simulink model "main"  (R2017b)
settings: Solver=FixedStepAuto  StartTime=0.0  StopTime=60  FixedStep=Ts  RelTol=1e-3
values from neighbouring files (symbols this model uses):
  ekfPendel = observer.formParameters()    [prepareWorkspace.m]
  Ts = 0.005    [prepareWorkspace.m]
undefined symbols (not defined in the file or in its folder): lambda, sigma, w0
libraries: hydro x2
settings Model: Creator=motionlab  LastModifiedBy=motionlab
settings OptimizationCC: LocalBlockOutputs=off
settings DebuggingCC: BusObjectLabelMismatch=error
settings SFSimCC: SimCustomHeaderCode=|
  | #include <ioTypes.h>
  | #include <simTypes.h>
  | #include <plcTypes.h>
settings RTWCC: SystemTargetFile=TwinCAT.tlc  GenCodeOnly=on  MakeCommand=make_tct  TemplateMakefile=tct_msbuild.tmf  Description=TwinCAT Target  GenerateReport=on  TargetLang=C++
settings STFCustomTargetCC: TargetLangStandard=C++03 (ISO)  CompOptLevelCompliant=on  MATLABClassNameForMDSCustomization=Simulink.SoftwareTarget.TargetSpecificTriggerConfigurationBase  SystemTargetFile=TwinCAT.tlc

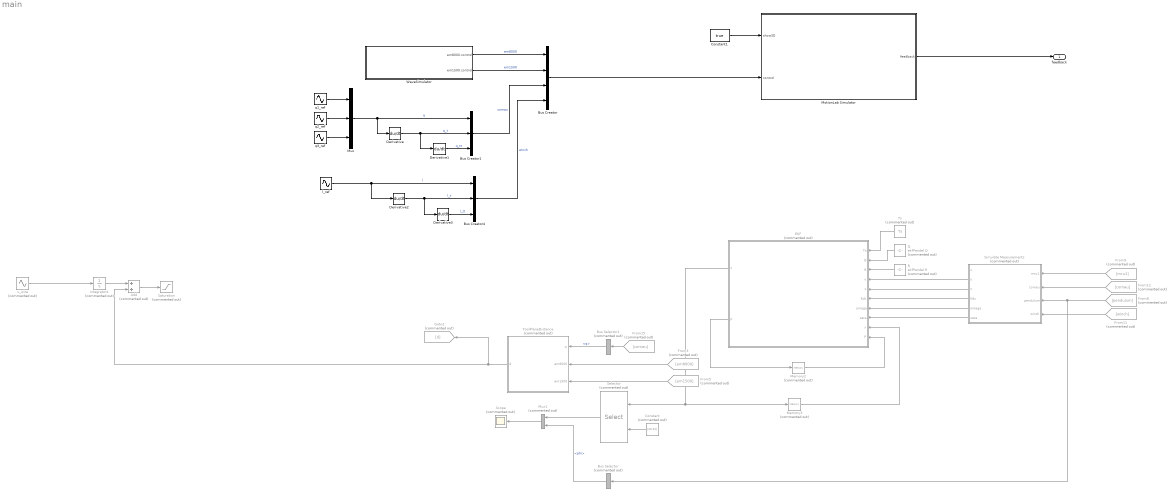
== system main ==
  Add : Sum  Commented=on
  Bus Creator : BusCreator  Inputs=4  OutDataTypeStr=Bus: ST_Control
  Bus Creator1 : BusCreator  Inputs=3  OutDataTypeStr=Bus: ST_ComauControl
  Bus Creator4 : BusCreator  Inputs=3  OutDataTypeStr=Bus: ST_WinchControl
  Bus Selector : BusSelector  Commented=on  OutputSignals=phi
  Bus Selector1 : BusSelector  Commented=on  OutputSignals=q
  Constant : Constant  Commented=on  Value=[30:31]
  Constant1 : Constant  Value=true
  Derivative{,1..3} (4 alike) : Derivative
  EKF : MATLAB Function  Commented=on  TreatAsAtomicUnit=on
  From11 : From  Commented=on  GotoTag=winch
  From12 : From  Commented=on  GotoTag=comau
  From15 : From  Commented=on  GotoTag=comau
  From3 : From  Commented=on  GotoTag=em8000
  From5 : From  Commented=on  GotoTag=em1500
  From8 : From  Commented=on  GotoTag=pendulum
  From9 : From  Commented=on  GotoTag=mru1
  Goto2 : Goto  Commented=on  GotoTag=d
  Integrator4 : Integrator  Commented=on
  Memory2 : Memory  Commented=on  InitialCondition=ekfPendel.P
  Memory3 : Memory  Commented=on  InitialCondition=ekfPendel.x0
  MotionLab Simulator : Subsystem
  Mux : Mux  Inputs=3
  Mux1 : Mux  Commented=on  Inputs=2
  Q : Constant  Commented=on  Value=ekfPendel.Q
  R : Constant  Commented=on  Value=ekfPendel.R
  Saturation : Saturate  Commented=on  UpperLimit=4.0  LowerLimit=0.5
  Scope : Scope  Commented=on
  Selector : Selector  Commented=on  InputPortWidth=34  IndexOptions=Index vector (port)  Indices=[1 3]  OutputSizes=1
  Simulate Measurements : MATLAB Function  Commented=on  TreatAsAtomicUnit=on
  ToolPlaneDistance : Subsystem  Commented=on  mask{d=-0.5}
      mask prompts: d "Plane-BodyOrigo Distance"
  Ts : Constant  Commented=on  Value=Ts
  WaveSimulator : Subsystem  mask{w0=w0, sigma=sigma, lambda=lambda}
      mask prompts: w0 "Peak Frequency"; sigma "Wave Intensity"; lambda "Damping"
  l_ref : Sin  Amplitude=0  Bias=2  Frequency=0.2*2*pi  SampleTime=0
  q1_ref : Sin  Amplitude=10/180*pi  Frequency=0.2*2*pi  SampleTime=0
  q2_ref : Sin  Amplitude=0  Frequency=0.1*2*pi  SampleTime=0
  q3_ref : Sin  Amplitude=0  Bias=-pi/2  Frequency=0.12*2*pi  SampleTime=0
  v_wire : Sin  Commented=on  Amplitude=0  Frequency=0.2*2*pi  SampleTime=0
  feedback : Outport
  wires:
  q2_ref/1 -> Mux/2
  q3_ref/1 -> Mux/3
  Mux/1 -> Bus Creator1/1, Derivative/1  "q"
  Derivative/1 -> Derivative1/1, Bus Creator1/2  "q_t"
  q1_ref/1 -> Mux/1
  Add/1 -> Saturation/1
  Integrator4/1 -> Add/1
  v_wire/1 -> Integrator4/1
  From3/1 -> ToolPlaneDistance/2(em8000)
  From5/1 -> ToolPlaneDistance/3(em1500)
  ToolPlaneDistance/1(d) -> Goto2/1, Add/2
  From12/1 -> Simulate Measurements/2(comau)
  From11/1 -> Simulate Measurements/4(winch)
  From9/1 -> Simulate Measurements/1(mru1)
  Ts/1 -> EKF/1(Ts)
  R/1 -> EKF/3(R)
  Simulate Measurements/6(zeta) -> EKF/8(zeta)
  Simulate Measurements/3(z) -> EKF/5(z)
  EKF/1(x) -> Memory3/1, Selector/1
  Memory3/1 -> EKF/9("x ")
  Q/1 -> EKF/2(Q)
  Simulate Measurements/2(u) -> EKF/4(u)
  Simulate Measurements/4(Kdc) -> EKF/6(Kdc)
  Memory2/1 -> EKF/10("P ")
  Selector/1 -> Mux1/1
  From8/1 -> Bus Selector/1, Simulate Measurements/3(pendulum)
  Simulate Measurements/5(omega) -> EKF/7(omega)
  Constant/1 -> Selector/2
  Mux1/1 -> Scope/1
  EKF/2(P) -> Memory2/1
  Bus Selector/1 -> Mux1/2  "<phi>"
  From15/1 -> Bus Selector1/1
  Bus Selector1/1 -> ToolPlaneDistance/1(q)  "<q>"
  Derivative1/1 -> Bus Creator1/3  "q_tt"
  Derivative2/1 -> Derivative3/1, Bus Creator4/2  "l_t"
  Derivative3/1 -> Bus Creator4/3  "l_tt"
  l_ref/1 -> Derivative2/1, Bus Creator4/1  "l"
  WaveSimulator/1(em8000.control) -> Bus Creator/1  "em8000"
  WaveSimulator/2(em1500.control) -> Bus Creator/2  "em1500"
  Bus Creator1/1 -> Bus Creator/3  "comau"
  Bus Creator4/1 -> Bus Creator/4  "winch"
  Bus Creator/1 -> MotionLab Simulator/2(control)
  MotionLab Simulator/1(feedback) -> feedback/1
  Constant1/1 -> MotionLab Simulator/1(show3D)

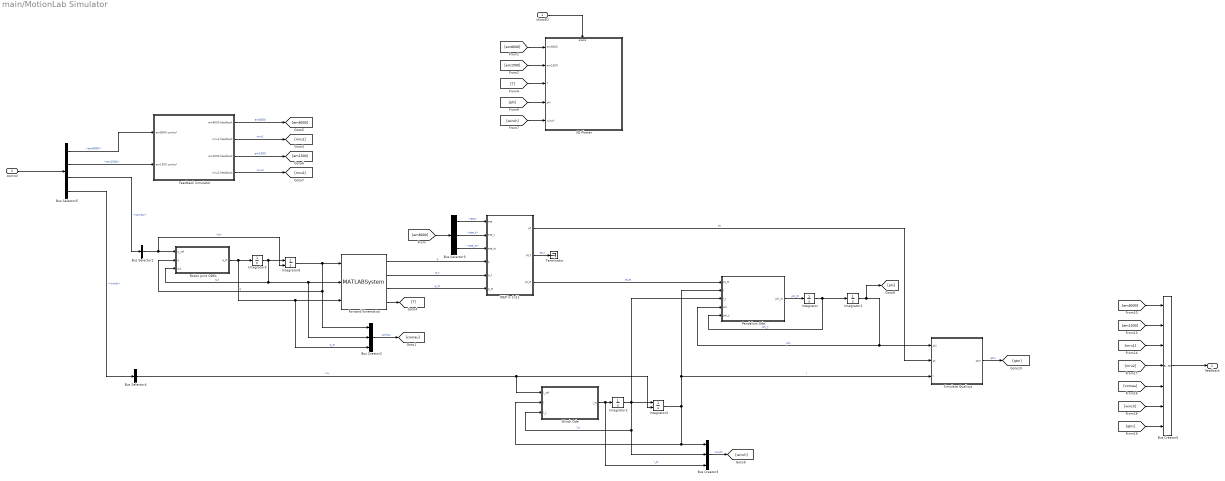
== system main/MotionLab Simulator ==
  show3D : Inport
  control : Inport  Port=2
  3D Plotter : Subsystem
  Bus Creator2 : BusCreator  Inputs=3  OutDataTypeStr=Bus: ST_ComauFeedback
  Bus Creator3 : BusCreator  Inputs=3  OutDataTypeStr=Bus: ST_WinchFeedback
  Bus Creator5 : BusCreator  Inputs=7  OutDataTypeStr=Bus: ST_Feedback
  Bus Selector2 : BusSelector  OutputSignals=q
  Bus Selector3 : BusSelector  OutputSignals=eta,eta_t,eta_tt
  Bus Selector4 : BusSelector  OutputSignals=l
  Bus Selector5 : BusSelector  OutputSignals=em8000,em1500,comau,winch
  Feedback Simulator : Subsystem
  Forward Kinematics : MATLABSystem  System=motionlab.ComauRobot3DOF  dt=L  fk=on  outputT=on  SimulateUsing=Interpreted execution
      mask Type: motionlab.ComauRobot3DOF
      mask Display:
      | disp('ComauRobot3DOF');
      | port_label('input',1,'q');
      | port_label('input',2,'q_t');
      | port_label('input',3,'q_tt');
      | port_label('output',1,'p');
      | port_label('output',2,'p_t');
      | port_label('output',3,'p_tt');
      | port_label('output',4,'T');
  Integrator : Integrator  InitialCondition=zeros(2,1)
  Integrator1 : Integrator  InitialCondition=zeros(2,1)
  Integrator2 : Integrator
  Integrator3 : Integrator  InitialConditionSource=external
  Integrator5 : Integrator  InitialCondition=zeros(3,1)
  Integrator6 : Integrator  InitialConditionSource=external  InitialCondition=zeros(3,1)
  Pendelum Ode : MATLAB Function  TreatAsAtomicUnit=on  SystemSampleTime=Ts
  Robot Joint ODEs : MATLAB Function  TreatAsAtomicUnit=on
  Simulate Qualisys : MATLAB Function  TreatAsAtomicUnit=on
  Terminator : Terminator
  "WEP in {n1}" : MATLAB Function  TreatAsAtomicUnit=on
  Winch Ode : MATLAB Function  TreatAsAtomicUnit=on
  feedback : Outport
  wires:
  [mru1] -> Bus Creator5/3
  [winch] -> 3D Plotter/5(winch)
  [mru2] -> Bus Creator5/4
  [em1500] -> Bus Creator5/2
  [em8000] -> Bus Creator5/1
  Bus Creator3/1 -> [winch]  "winch"
  Bus Creator5/1 -> feedback/1
  [qtm] -> Bus Creator5/7
  [comau] -> Bus Creator5/5
  [winch] -> Bus Creator5/6
  "WEP in {n1}"/2(pt_t) -> Terminator/1  "pt_t"
  Winch Ode/1(l_tt) -> Bus Creator3/3, Integrator2/1  "l_tt"
  show3D/1 -> 3D Plotter/Enable
  Integrator/1 -> Integrator1/1, Pendelum Ode/5(phi_t)  "phi_t"
  "WEP in {n1}"/3(pt_tt) -> Pendelum Ode/1(pt_tt)  "pt_tt"
  Forward Kinematics/4 -> [T]
  Bus Selector2/1 -> Robot Joint ODEs/1(q_ref), Integrator6/2  "<q>"
  Pendelum Ode/1(phi_tt) -> Integrator/1  "phi_tt"
  Integrator3/1 -> Winch Ode/2(l), Bus Creator3/1, Pendelum Ode/2(l), Simulate Qualisys/3(l)  "l"
  Integrator2/1 -> Pendelum Ode/3(l_t), Bus Creator3/2, Winch Ode/3(l_t), Integrator3/1  "l_t"
  Integrator1/1 -> [phi], Pendelum Ode/4(phi), Simulate Qualisys/1(phi)  "phi"
  Robot Joint ODEs/1(q_tt) -> Integrator5/1, Bus Creator2/3, Forward Kinematics/3  "q_tt"
  Integrator5/1 -> Robot Joint ODEs/3(q_t), Forward Kinematics/2, Bus Creator2/2, Integrator6/1  "q_t"
  Integrator6/1 -> Bus Creator2/1, Robot Joint ODEs/2(q), Forward Kinematics/1  "q"
  Forward Kinematics/1 -> "WEP in {n1}"/4(p)  "p"
  Forward Kinematics/2 -> "WEP in {n1}"/5(p_t)  "p_t"
  Forward Kinematics/3 -> "WEP in {n1}"/6(p_tt)  "p_tt"
  Simulate Qualisys/1(qtm) -> [qtm]  "qtm"
  Bus Selector4/1 -> Winch Ode/1(l_ref), Integrator3/2  "<l>"
  control/1 -> Bus Selector5/1
  Bus Selector5/1 -> Feedback Simulator/1(em8000.control)  "<em8000>"
  Bus Selector3/1 -> "WEP in {n1}"/1(eta)  "<eta>"
  Bus Selector3/3 -> "WEP in {n1}"/3(eta_tt)  "<eta_tt>"
  Bus Selector3/2 -> "WEP in {n1}"/2(eta_t)  "<eta_t>"
  "WEP in {n1}"/1(pt) -> Simulate Qualisys/2(pt)  "pt"
  Bus Selector5/2 -> Feedback Simulator/2(em1500.control)  "<em1500>"
  Feedback Simulator/1(em8000.feedback) -> [em8000]  "em8000"
  [phi] -> 3D Plotter/4(phi)
  Feedback Simulator/3(em1500.feedback) -> [em1500]  "em1500"
  [em8000] -> Bus Selector3/1
  [em1500] -> 3D Plotter/2(em1500)
  Feedback Simulator/2(mru1.feedback) -> [mru1]  "mru1"
  Bus Selector5/3 -> Bus Selector2/1  "<comau>"
  [em8000] -> 3D Plotter/1(em8000)
  Bus Creator2/1 -> [comau]  "comau"
  Feedback Simulator/4(mru2.feedback) -> [mru2]  "mru2"
  Bus Selector5/4 -> Bus Selector4/1  "<winch>"
  [T] -> 3D Plotter/3(T)

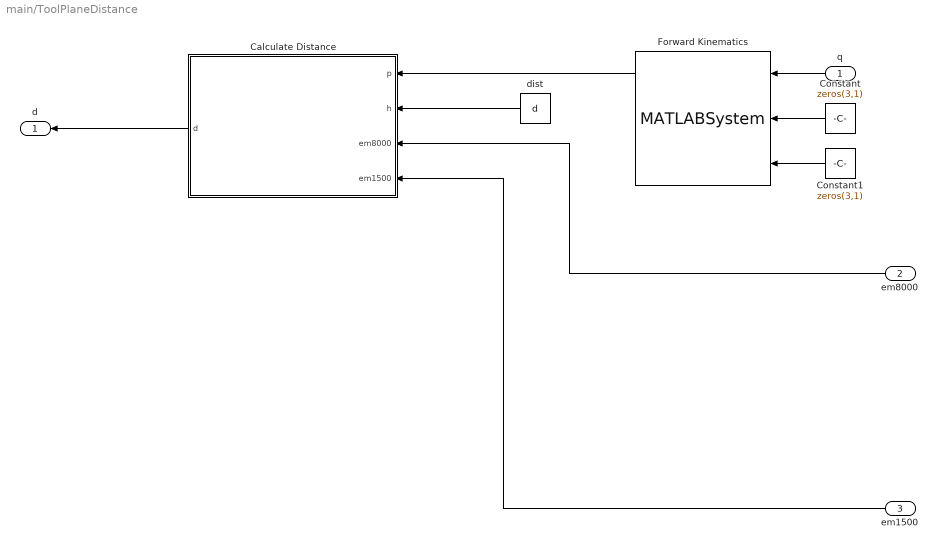
== system main/ToolPlaneDistance ==
  q : Inport
  em8000 : Inport  Port=2  OutDataTypeStr=Bus: StewartFeedback
  em1500 : Inport  Port=3  OutDataTypeStr=Bus: StewartFeedback
  Calculate Distance : MATLAB Function  TreatAsAtomicUnit=on
  Constant : Constant  Value=zeros(3,1)
  Constant1 : Constant  Value=zeros(3,1)
  Forward Kinematics : MATLABSystem  System=motionlab.ComauRobot3DOF  dt=L  fk=on  outputT=off  SimulateUsing=Interpreted execution
      mask Type: motionlab.ComauRobot3DOF
      mask Display:
      | disp('ComauRobot3DOF');
      | port_label('input',1,'q');
      | port_label('input',2,'q_t');
      | port_label('input',3,'q_tt');
      | port_label('output',1,'p');
      | port_label('output',2,'p_t');
      | port_label('output',3,'p_tt');
  dist : Constant  Value=d
  d : Outport
  wires:
  Calculate Distance/1(d) -> d/1
  Constant/1 -> Forward Kinematics/2
  Constant1/1 -> Forward Kinematics/3
  dist/1 -> Calculate Distance/2(h)
  em1500/1 -> Calculate Distance/4(em1500)
  em8000/1 -> Calculate Distance/3(em8000)
  Forward Kinematics/1 -> Calculate Distance/1(p)
  q/1 -> Forward Kinematics/1

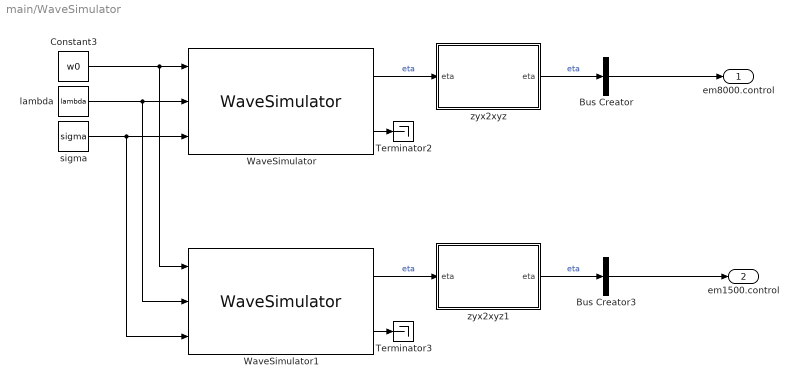
== system main/WaveSimulator ==
  Bus Creator : BusCreator  Inputs=1  OutDataTypeStr=Bus: ST_StewartControl
  Bus Creator3 : BusCreator  Inputs=1  OutDataTypeStr=Bus: ST_StewartControl
  Constant3 : Constant  Value=w0
  Terminator2 : Terminator
  Terminator3 : Terminator
  WaveSimulator : hydro/WaveSimulator  poles=-30  seed=[0,20,510,9000,400,200]  K1=1e4  K2=1e4  K3=1e8  K4=1e7  K5=1e8  K6=1e3  maxOutput=[0.2, 0.2, 0.4, 10/180*pi, 10/180*pi, 5/180*pi]  limitK=[1, 1, 0.15, 1, 1, 1]
      settings: SourceProductName=Hydro Library
  WaveSimulator1 : hydro/WaveSimulator  poles=-30  seed=[5000,400,0,9000,150,42]  K1=1e4  K2=1e4  K3=1e8  K4=1e7  K5=1e8  K6=1e3  maxOutput=[0.2, 0.2, 0.4, 5/180*pi, 5/180*pi, 5/180*pi]  limitK=[1, 1, 0.15, 1, 1, 1]
      settings: SourceProductName=Hydro Library
  lambda : Constant  Value=lambda
  sigma : Constant  Value=sigma
  zyx2xyz : MATLAB Function  TreatAsAtomicUnit=on
  zyx2xyz1 : MATLAB Function  TreatAsAtomicUnit=on
  em8000.control : Outport
  em1500.control : Outport  Port=2
  wires:
  zyx2xyz/1(eta) -> Bus Creator/1  "eta"
  Bus Creator3/1 -> em1500.control/1
  Bus Creator/1 -> em8000.control/1
  zyx2xyz1/1(eta) -> Bus Creator3/1  "eta"
  sigma/1 -> WaveSimulator1/3, WaveSimulator/3
  Constant3/1 -> WaveSimulator1/1, WaveSimulator/1
  WaveSimulator1/1 -> zyx2xyz1/1("eta ")  "eta"
  WaveSimulator/2 -> Terminator2/1
  WaveSimulator/1 -> zyx2xyz/1("eta ")  "eta"
  lambda/1 -> WaveSimulator1/2, WaveSimulator/2
  WaveSimulator1/2 -> Terminator3/1

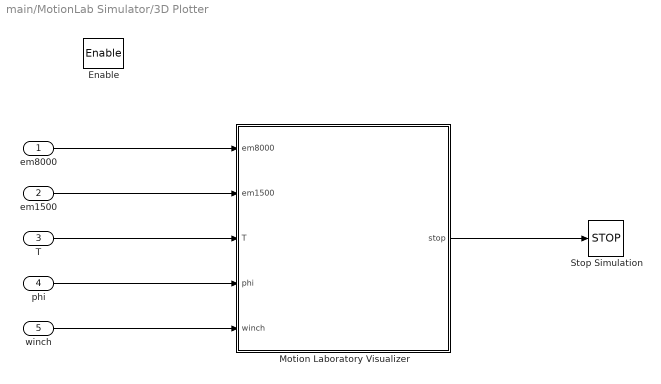
== system main/MotionLab Simulator/3D Plotter ==
  em8000 : Inport
  em1500 : Inport  Port=2
  T : Inport  Port=3
  phi : Inport  Port=4
  winch : Inport  Port=5
  Enable : EnablePort
  Motion Laboratory Visualizer : MATLAB Function  TreatAsAtomicUnit=on  SystemSampleTime=0.1
  Stop Simulation : Stop
  wires:
  em8000/1 -> Motion Laboratory Visualizer/1(em8000)
  phi/1 -> Motion Laboratory Visualizer/4(phi)
  winch/1 -> Motion Laboratory Visualizer/5(winch)
  em1500/1 -> Motion Laboratory Visualizer/2(em1500)
  T/1 -> Motion Laboratory Visualizer/3(T)
  Motion Laboratory Visualizer/1(stop) -> Stop Simulation/1

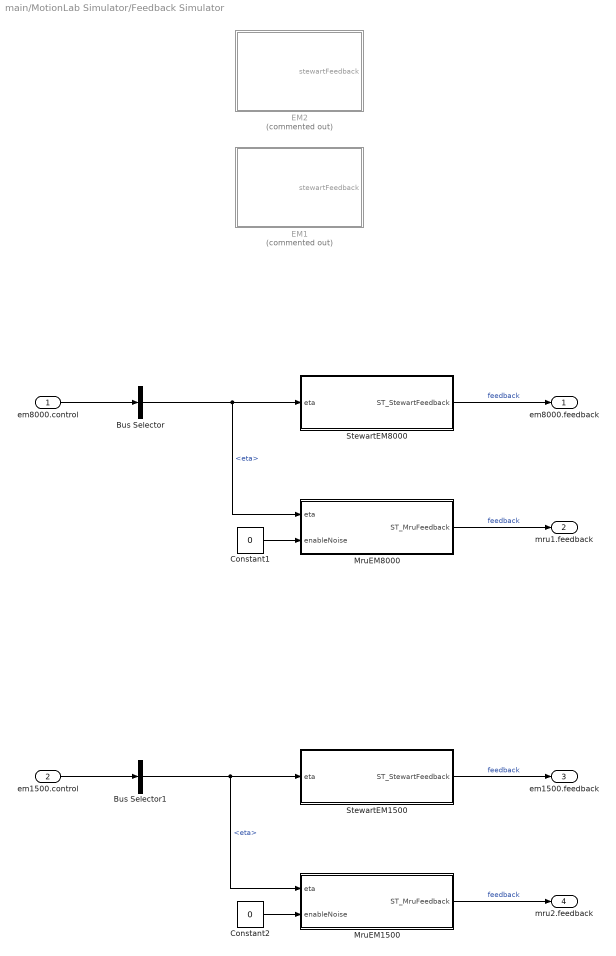
== system main/MotionLab Simulator/Feedback Simulator ==
  em8000.control : Inport  OutDataTypeStr=Bus: ST_StewartControl
  em1500.control : Inport  Port=2  OutDataTypeStr=Bus: ST_StewartControl
  Bus Selector : BusSelector  OutputSignals=eta
  Bus Selector1 : BusSelector  OutputSignals=eta
  Constant1 : Constant  Value=0
  Constant2 : Constant  Value=0
  EM1 : Subsystem  Commented=on  TreatAsAtomicUnit=on  mask{A_surge=0.2, f_surge=0.1, phase_surge=0, A_sway=0.2, f_sway=0.05, phase_sway=200, A_heave=0.4, f_heave=0.12, phase_heave=30, A_phi=5.0, f_phi=0.09, phase_phi=45, A_theta=5.0, f_theta=0.15, phase_theta=60, A_psi=5.0, f_psi=0.12, phase_psi=-40}
      mask prompts: A_surge "Amplitude [m]"; f_surge "Frequency [Hz]"; phase_surge "Phase [deg]"; A_sway "Amplitude [m]"; f_sway "Frequency [Hz]"; phase_sway "Phase [deg]"; A_heave "Amplitude [m]"; f_heave "Frequency [Hz]"; phase_heave "Phase [deg]"; A_phi "Amplitude [deg]"; f_phi "Frequency [Hz]"; phase_phi "Phase [deg]"; A_theta "Amplitude [deg]"; f_theta "Frequency [Hz]"; phase_theta "Phase [deg]"; A_psi "Amplitude [deg]"; f_psi "Frequency [Hz]"; phase_psi "Phase [deg]"
      mask DialogControl ParameterGroupVar Prompt: Surge
      mask DialogControl Container3 Prompt: Sway
      mask DialogControl Container4 Prompt: Heave
      mask DialogControl Container5 Prompt: Phi
      mask DialogControl Container6 Prompt: Theta
      mask DialogControl Container7 Prompt: Psi
  EM2 : Subsystem  Commented=on  TreatAsAtomicUnit=on  mask{A_surge=0.05, f_surge=0.1, phase_surge=0, A_sway=0.05, f_sway=0.12, phase_sway=120, A_heave=0.4, f_heave=0.12, phase_heave=30, A_phi=5, f_phi=0.09, phase_phi=45, A_theta=5, f_theta=0.15, phase_theta=60, A_psi=5, f_psi=0.12, phase_psi=-40}
      mask prompts: A_surge "Amplitude [m]"; f_surge "Frequency [Hz]"; phase_surge "Phase [deg]"; A_sway "Amplitude [m]"; f_sway "Frequency [Hz]"; phase_sway "Phase [deg]"; A_heave "Amplitude [m]"; f_heave "Frequency [Hz]"; phase_heave "Phase [deg]"; A_phi "Amplitude [deg]"; f_phi "Frequency [Hz]"; phase_phi "Phase [deg]"; A_theta "Amplitude [deg]"; f_theta "Frequency [Hz]"; phase_theta "Phase [deg]"; A_psi "Amplitude [deg]"; f_psi "Frequency [Hz]"; phase_psi "Phase [deg]"
      mask DialogControl ParameterGroupVar Prompt: Surge
      mask DialogControl Container3 Prompt: Sway
      mask DialogControl Container4 Prompt: Heave
      mask DialogControl Container5 Prompt: Phi
      mask DialogControl Container6 Prompt: Theta
      mask DialogControl Container7 Prompt: Psi
  MruEM1500 : Subsystem
  MruEM8000 : Subsystem
  StewartEM1500 : Subsystem
  StewartEM8000 : Subsystem
  em8000.feedback : Outport
  mru1.feedback : Outport  Port=2
  em1500.feedback : Outport  Port=3
  mru2.feedback : Outport  Port=4
  wires:
  Constant1/1 -> MruEM8000/2(enableNoise)
  Constant2/1 -> MruEM1500/2(enableNoise)
  StewartEM8000/1(ST_StewartFeedback) -> em8000.feedback/1  "feedback"
  MruEM8000/1(ST_MruFeedback) -> mru1.feedback/1  "feedback"
  StewartEM1500/1(ST_StewartFeedback) -> em1500.feedback/1  "feedback"
  MruEM1500/1(ST_MruFeedback) -> mru2.feedback/1  "feedback"
  em8000.control/1 -> Bus Selector/1
  Bus Selector/1 -> MruEM8000/1(eta), StewartEM8000/1(eta)  "<eta>"
  em1500.control/1 -> Bus Selector1/1
  Bus Selector1/1 -> MruEM1500/1(eta), StewartEM1500/1(eta)  "<eta>"

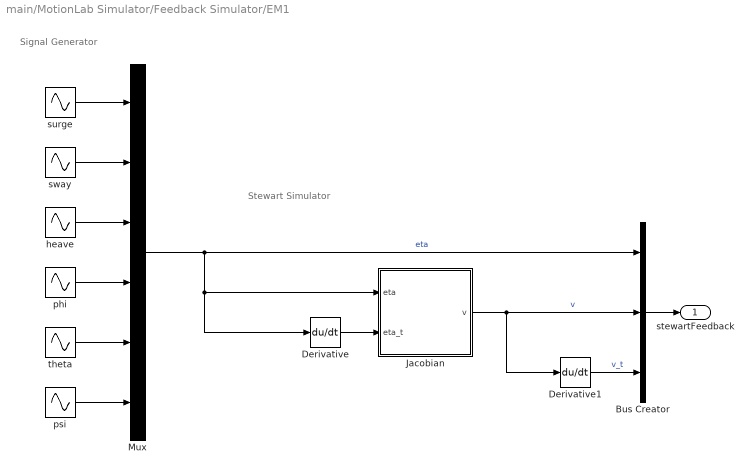
== system main/MotionLab Simulator/Feedback Simulator/EM1 ==
  note: Signal Generator
  note: Stewart Simulator
  Bus Creator : BusCreator  Inputs=3  OutDataTypeStr=Bus: StewartFeedback
  Derivative : Derivative
  Derivative1 : Derivative
  Jacobian : MATLAB Function  TreatAsAtomicUnit=on
  Mux : Mux  Inputs=6
  heave : Sin  Amplitude=A_heave  Frequency=f_heave*2*pi  Phase=phase_heave/180*pi
  phi : Sin  Amplitude=A_phi/180*pi  Frequency=f_phi*2*pi  Phase=phase_phi/180*pi
  psi : Sin  Amplitude=A_psi/180*pi  Frequency=f_psi*2*pi  Phase=phase_psi/180*pi
  surge : Sin  Amplitude=A_surge  Frequency=f_surge*2*pi  Phase=phase_surge/180*pi
  sway : Sin  Amplitude=A_sway  Frequency=f_sway*2*pi  Phase=phase_sway/180*pi
  theta : Sin  Amplitude=A_theta/180*pi  Frequency=f_theta*2*pi  Phase=phase_theta/180*pi
  stewartFeedback : Outport  OutDataTypeStr=Bus: StewartFeedback
  wires:
  psi/1 -> Mux/6
  phi/1 -> Mux/4
  sway/1 -> Mux/2
  theta/1 -> Mux/5
  surge/1 -> Mux/1
  heave/1 -> Mux/3
  Jacobian/1(v) -> Derivative1/1, Bus Creator/2  "v"
  Mux/1 -> Bus Creator/1, Derivative/1, Jacobian/1(eta)  "eta"
  Derivative/1 -> Jacobian/2(eta_t)
  Derivative1/1 -> Bus Creator/3  "v_t"
  Bus Creator/1 -> stewartFeedback/1

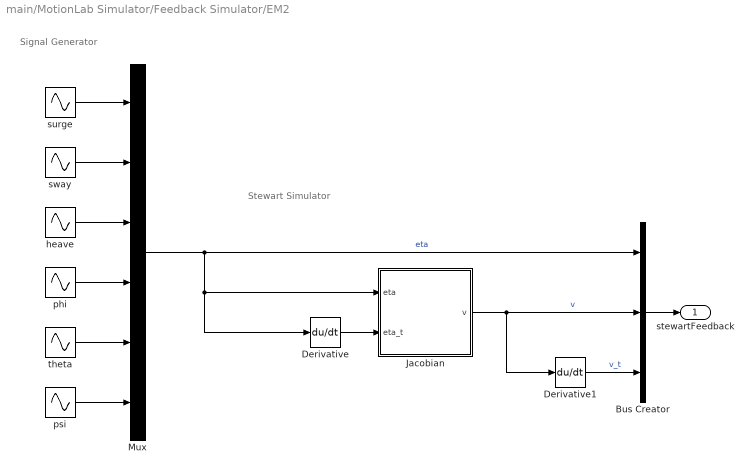
== system main/MotionLab Simulator/Feedback Simulator/EM2 ==
  note: Signal Generator
  note: Stewart Simulator
  Bus Creator : BusCreator  Inputs=3  OutDataTypeStr=Bus: StewartFeedback
  Derivative : Derivative
  Derivative1 : Derivative  CoefficientInTFapproximation=-1
  Jacobian : MATLAB Function  TreatAsAtomicUnit=on
  Mux : Mux  Inputs=6
  heave : Sin  Amplitude=A_heave  Frequency=f_heave*2*pi  Phase=phase_heave/180*pi
  phi : Sin  Amplitude=A_phi/180*pi  Frequency=f_phi*2*pi  Phase=phase_phi/180*pi
  psi : Sin  Amplitude=A_psi/180*pi  Frequency=f_psi*2*pi  Phase=phase_psi/180*pi
  surge : Sin  Amplitude=A_surge  Frequency=f_surge*2*pi  Phase=phase_surge/180*pi
  sway : Sin  Amplitude=A_sway  Frequency=f_sway*2*pi  Phase=phase_sway/180*pi
  theta : Sin  Amplitude=A_theta/180*pi  Frequency=f_theta*2*pi  Phase=phase_theta/180*pi
  stewartFeedback : Outport  OutDataTypeStr=Bus: StewartFeedback
  wires:
  psi/1 -> Mux/6
  phi/1 -> Mux/4
  sway/1 -> Mux/2
  theta/1 -> Mux/5
  surge/1 -> Mux/1
  heave/1 -> Mux/3
  Jacobian/1(v) -> Derivative1/1, Bus Creator/2  "v"
  Mux/1 -> Bus Creator/1, Derivative/1, Jacobian/1(eta)  "eta"
  Derivative/1 -> Jacobian/2(eta_t)
  Derivative1/1 -> Bus Creator/3  "v_t"
  Bus Creator/1 -> stewartFeedback/1

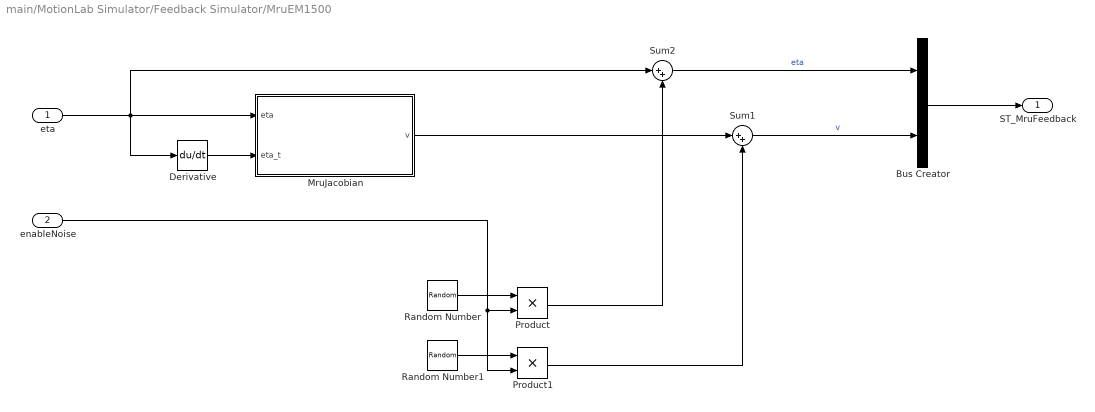
== system main/MotionLab Simulator/Feedback Simulator/MruEM1500 ==
  eta : Inport
  enableNoise : Inport  Port=2
  Bus Creator : BusCreator  Inputs=2  OutDataTypeStr=Bus: ST_MruFeedback
  Derivative : Derivative
  MruJacobian : MATLAB Function  TreatAsAtomicUnit=on
  Product : Product
  Product1 : Product
  Random Number : RandomNumber  Variance=sim.mru1.var.eta  Seed=randi(100000, 6, 1)  SampleTime=Ts
  Random Number1 : RandomNumber  Variance=sim.mru1.var.v  Seed=randi(100000, 6, 1)  SampleTime=Ts
  Sum1 : Sum  Inputs=|++
  Sum2 : Sum  Inputs=|++
  ST_MruFeedback : Outport  OutDataTypeStr=Bus: ST_MruFeedback
  wires:
  Derivative/1 -> MruJacobian/2(eta_t)
  eta/1 -> Sum2/1, Derivative/1, MruJacobian/1(eta)
  MruJacobian/1(v) -> Sum1/1
  Sum1/1 -> Bus Creator/2  "v"
  Sum2/1 -> Bus Creator/1  "eta"
  Random Number/1 -> Product/1
  Product/1 -> Sum2/2
  Random Number1/1 -> Product1/1
  Product1/1 -> Sum1/2
  enableNoise/1 -> Product1/2, Product/2
  Bus Creator/1 -> ST_MruFeedback/1

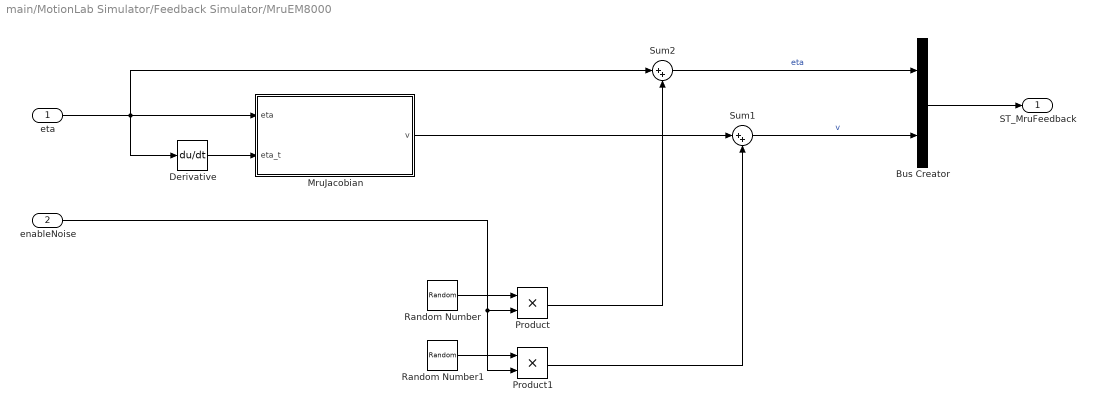
== system main/MotionLab Simulator/Feedback Simulator/MruEM8000 ==
  eta : Inport
  enableNoise : Inport  Port=2
  Bus Creator : BusCreator  Inputs=2  OutDataTypeStr=Bus: ST_MruFeedback
  Derivative : Derivative
  MruJacobian : MATLAB Function  TreatAsAtomicUnit=on
  Product : Product
  Product1 : Product
  Random Number : RandomNumber  Variance=sim.mru1.var.eta  Seed=randi(100000, 6, 1)  SampleTime=Ts
  Random Number1 : RandomNumber  Variance=sim.mru1.var.v  Seed=randi(100000, 6, 1)  SampleTime=Ts
  Sum1 : Sum  Inputs=|++
  Sum2 : Sum  Inputs=|++
  ST_MruFeedback : Outport  OutDataTypeStr=Bus: ST_MruFeedback
  wires:
  Derivative/1 -> MruJacobian/2(eta_t)
  eta/1 -> Sum2/1, Derivative/1, MruJacobian/1(eta)
  MruJacobian/1(v) -> Sum1/1
  Sum1/1 -> Bus Creator/2  "v"
  Sum2/1 -> Bus Creator/1  "eta"
  Random Number/1 -> Product/1
  Product/1 -> Sum2/2
  Random Number1/1 -> Product1/1
  Product1/1 -> Sum1/2
  enableNoise/1 -> Product1/2, Product/2
  Bus Creator/1 -> ST_MruFeedback/1

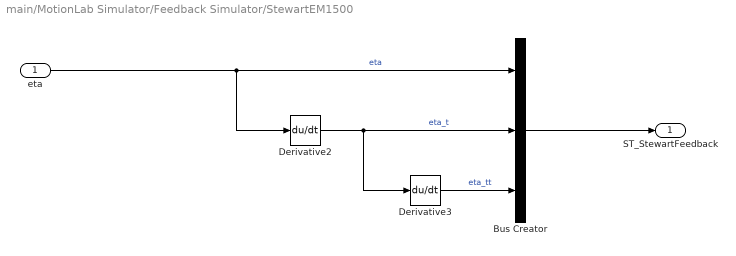
== system main/MotionLab Simulator/Feedback Simulator/StewartEM1500 ==
  eta : Inport
  Bus Creator : BusCreator  Inputs=3  OutDataTypeStr=Bus: ST_StewartFeedback
  Derivative2 : Derivative
  Derivative3 : Derivative  CoefficientInTFapproximation=-1
  ST_StewartFeedback : Outport  OutDataTypeStr=Bus: ST_StewartFeedback
  wires:
  Derivative2/1 -> Bus Creator/2, Derivative3/1  "eta_t"
  Bus Creator/1 -> ST_StewartFeedback/1
  Derivative3/1 -> Bus Creator/3  "eta_tt"
  eta/1 -> Bus Creator/1, Derivative2/1  "eta"

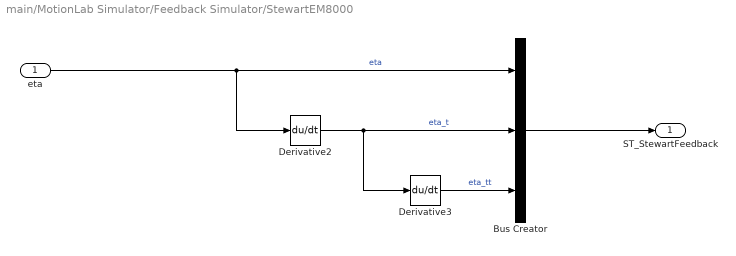
== system main/MotionLab Simulator/Feedback Simulator/StewartEM8000 ==
  eta : Inport
  Bus Creator : BusCreator  Inputs=3  OutDataTypeStr=Bus: ST_StewartFeedback
  Derivative2 : Derivative
  Derivative3 : Derivative  CoefficientInTFapproximation=-1
  ST_StewartFeedback : Outport  OutDataTypeStr=Bus: ST_StewartFeedback
  wires:
  Derivative2/1 -> Bus Creator/2, Derivative3/1  "eta_t"
  Bus Creator/1 -> ST_StewartFeedback/1
  Derivative3/1 -> Bus Creator/3  "eta_tt"
  eta/1 -> Bus Creator/1, Derivative2/1  "eta"

== matlab function main/MotionLab Simulator/3D Plotter/Motion Laboratory Visualizer ==
  data: stop output; em8000 input; em1500 input; T input; phi input; winch input
function stop  = fcn(em8000, em1500, T, phi, winch)

% Load calibration data
coderData = coder.load('+motionlab/calib.mat');
calib = coderData.calib;

% Load plot objects
%sphere = coder.load('spherePatch.mat');


% {g} -> {b1}
H1 = eye(4);
H1(1:3,4)= em8000.eta(1:3);
H1(1:3,1:3) = math3d.Rxyz(em8000.eta(4:6));

Hgn1 = calib.WORLD_TO_EM8000.H;
Hgb1 = Hgn1*H1;

% {g} -> {b2}
H2 = eye(4);
H2(1:3,4)= em1500.eta(1:3);
H2(1:3,1:3) = math3d.Rxyz(em1500.eta(4:6));

Hgn2 = calib.WORLD_TO_EM1500.H;
Hgb2 = Hgn2*H2;

% {b1} -> {r}
H1r = calib.EM8000_TO_COMAU.H;

% {r} -> {j1}
Hr1 = T(:,:,1);
Hr2 = Hr1*T(:,:,2);
Hr3 = Hr2*T(:,:,3);
Hrt = Hr3*T(:,:,4);



% Set up plot
persistent h;

% Declare plot3 as extrinsic
coder.extrinsic('plot3');


if isempty(h)
    close all
    
    h = figure('Name', 'Animation');
    hold on;
    grid on;
    axis equal;
    view([-40, 20]);
    
    
    % View limits
    xlim([-4, 2])
    ylim([-3, 3])
    zlim([0, 7])
    
    % Labels
    xlabel('x-axis')
    ylabel('y-axis')
    zlabel('z-axis')
    
    % Figure sizing
    screeenSz = [1920, 1200];
    figSz = [4, 3]/4*1200;
    set(h, 'Position', [
        screeenSz(1)/2 - figSz(1)/2
        screeenSz(2)/2 - figSz(2)/2
        figSz(1)
        figSz(2)
    ])
end

if ishandle(h)
    cla;
    
    % Ground coordinate system
    plotCoordinateSystem(eye(4));
    
    % EM8000
    plotCoordinateSystem(Hgn1);
    plotCoordinateSystem(Hgb1);
    
    % EM1500
    plotCoordinateSystem(Hgn2);
    plotCoordinateSystem(Hgb2);
    
    % Comau Robot Coordinates given in {g}
    Hgr = Hgb1*H1r;
    Hg1 = Hgr*Hr1;
    Hg2 = Hgr*Hr2;
    Hg3 = Hgr*Hr3;
    Hgt = Hgr*Hrt;
    
    Hgq = calib.WORLD_TO_QTM.H;
    
    % Hook position in {n1}   
    pt_n = Hgn1(1:3,1:3)'*Hgt(1:3,4);
    ph_n = pendel.kinematics(pt_n, phi, winch.l);
    
    ph = Hgn1(1:3,1:3)*ph_n;
    
    % Robot Coordinates
    plotCoordinateSystem(Hgr);
    plotCoordinateSystem(Hg1);
    plotCoordinateSystem(Hg2);
    plotCoordinateSystem(Hg3);
    plotCoordinateSystem(Hgt);
    
    % Qualisys coordinate
    plotCoordinateSystem(Hgq);
    
    % Links
    plotLine(Hgr(1:3,4), Hg1(1:3,4));
    plotLine(Hg1(1:3,4), Hg2(1:3,4));
    plotLine(Hg2(1:3,4), Hg3(1:3,4));
    plotLine(Hg3(1:3,4), Hgt(1:3,4));
    
    % Load
    plotLine(Hgt(1:3,4), ph);
    %plotLoadSphere(ph, sphere.fvc);
    
    % Plot ship plane
    plotPlane(Hgb2);
    
%     % Projected point
%     Hn1t = math3d.InvH(Hgn1)*Hgt;
%     dir = [0; 0; 1];
%     pp = Hn1t(1:3,4) + d*dir;
%     p = Hgn1*[pp; 1];
%     plot3(p(1), p(2), p(3), 'k.')
    
      
    % Update plots
    drawnow;
end


% Close when figure is closed
stop = false;
if ~ishandle(h)
    stop = true;
end



end

function plotLine(p1, p2)
    link = zeros(2,3);
    link(1,:) = p1;
    link(2,:) = p2;
    
    plot3(link(:,1), link(:,2), link(:,3), 'k')
end

function plotLoadSphere(ph, fvc)
    coder.extrinsic('patch');

    % Patch data
    fvc.vertices(:,1) = fvc.vertices(:,1) + ph(1);
    fvc.vertices(:,2) = fvc.vertices(:,2) + ph(2);
    fvc.vertices(:,3) = fvc.vertices(:,3) + ph(3);
    
    patch('Faces', fvc.faces, 'Vertices', fvc.vertices, 'FaceColor', 'k')
    
end

function plotPlane(H)

coder.extrinsic('patch');

x = 3/2;
y = 5/2;
z = -0.5;
xyPlane = [
    -x,  x,  x, -x
    -y, -y,  y,  y
     z,  z,  z,  z
     1,  1,  1,  1
];

plane = H*xyPlane;

patch(plane(1,:), plane(2,:), plane(3,:), 'r', 'FaceAlpha', 0.5);

end

function plotCoordinateSystem(varargin)
    % Rotation and translation
    H = varargin{1};
    t = H(1:3,4);
    R = H(1:3,1:3);

    % Axis colors
    colors = {'r', 'g', 'b'};

    % Plot all 3 axis
    axis = zeros(2,3);
    axLength = 0.4;
    for i = 1:3
        axis(1,:) = t;
        axis(2,:) = t + R(:,i)*axLength;

        plot3(axis(:,1), axis(:,2), axis(:,3), colors{i}, 'LineWidth', 1);
    end
    
    if nargin > 1
        loc = mean(axis);
        text(loc(1), loc(2), loc(3), varargin{2})
    end
end

== matlab function main/WaveSimulator/zyx2xyz ==
  data: eta input; eta output
function eta = fcn(eta)

% Convert Angle sequence
eta(4:6) = math3d.zyx2xyz(eta(4:6));

end

== matlab function main/MotionLab Simulator/Feedback Simulator/MruEM1500/MruJacobian ==
  data: eta input; v output; eta_t input
function v = fcn(eta, eta_t)

% Velcoity Jacobian
J = eye(6);
J(4:6,4:6) = math3d.Tphi(eta(4:6), 'xyz');

% Body fixed velocities
v = J\eta_t;

end

== matlab function main/MotionLab Simulator/Pendelum Ode ==
  data: phi_tt output; pt_tt input; l input; l_t input; phi input; phi_t input
function phi_tt  = fcn(pt_tt, l, l_t, phi, phi_t)
% Paramaters
g = 9.81;
c = 0.2;

phi_tt = pendel.ode(phi, phi_t, pt_tt, l, l_t, g);

% add friction to pendulum
phi_tt = phi_tt - c*phi_t;

end

== matlab function main/MotionLab Simulator/WEP in {n1} ==
  data: eta input; eta_t input; pt output; pt_t output; pt_tt output; eta_tt input; p input; p_t input; p_tt input
function [pt, pt_t, pt_tt] = fcn(eta, eta_t, eta_tt, p, p_t, p_tt)
    
    % Get body velocites
    [v, v_t] = math3d.eulerToBody(eta, eta_t, eta_tt, 'xyz');

    % Load Calibration data
    data = coder.load('motionlab/calib.mat');
    calib = data.calib;
    
    % Robot pose relative to EM8000
    Hbr = calib.EM8000_TO_COMAU.H;

    % Ship/stewart {b} orientation matrix relative to {n}
    Rnb = math3d.Rxyz(eta(4:6));

    % Body fixed velocity and acceleration skew matrices
    W = math3d.skew(v(4:6));
    W_t = math3d.skew(v_t(4:6));

    Rnb_t = Rnb*W;
    Rnb_tt = Rnb*W*W + Rnb*W_t;

    % Constant offsets {b} -> {r}
    r = Hbr(1:3,4);
    Rbr = Hbr(1:3,1:3);

    % Position of {t}/{n} given in {n}
    pt = eta(1:3) + Rnb*(r + Rbr*p);

    % Velocity of {t}/{n} given in {n}
    pt_t = v(1:3) + Rnb_t*(r + Rbr*p) + Rnb*(Rbr*p_t);

    % Acceleration of {t}/{n} given in {n}
    pt_tt = v_t(1:3) + Rnb_tt*(r + Rbr*p)...
        + 2*Rnb_t*(Rbr*p_t) + Rnb*(Rbr*p_tt);
end

== matlab function main/MotionLab Simulator/Winch Ode ==
  data: l_ref input; l_tt output; l input; l_t input
function l_tt  = fcn(l_ref, l, l_t)

Kdc = 1.0;
omega = 4*2*pi;
zeta = 0.7;

l_tt = l_ref*Kdc*omega^2 - 2*zeta*omega*l_t - omega^2*l;
end

== matlab function main/MotionLab Simulator/Robot Joint ODEs ==
  data: q_ref input; q_tt output; q input; q_t input
function q_tt = fcn(q_ref, q, q_t)

Kdc = 1.0;
w = 10*2*pi;
zeta = 0.7;

q_tt = q_ref*Kdc*w^2 - 2*zeta*w*q_t - w^2*q;


end

== matlab function main/ToolPlaneDistance/Calculate Distance ==
  data: p input; h input; em8000 input; em1500 input; d output
function d  = fcn(p, h, em8000, em1500)

% Vectorize data
eta1 = [
    em8000.surge
    em8000.sway
    em8000.heave
    em8000.phi
    em8000.theta
    em8000.psi
];

eta2 = [
    em1500.surge
    em1500.sway
    em1500.heave
    em1500.phi
    em1500.theta
    em1500.psi
];

% Load calibration data
data = coder.load('motionlab/calib.mat');

H_b1r = data.calib.EM8000_TO_COMAU.H;

r1 = eta1(1:3);
Rn1b1 = math3d.Rxyz(eta1(4:6));

% {t}/{n1} given in {n1}
pt = r1 + Rn1b1*(H_b1r(1:3,4) + H_b1r(1:3,1:3)*p);

% Get plane normal vecotr of secondary ship
Hn1n2 = data.calib.EM8000_TO_EM1500.H;

Hn2b2 = eye(4);
Hn2b2(1:3,4) = eta2(1:3);
Hn2b2(1:3,1:3) = math3d.Rxyz(eta2(4:6));

Hn1b2 = Hn1n2*Hn2b2;

P0 = Hn1b2*[0; 0; h; 1];

% Use Line-Plane projection to get point laying on the ship plane
% http://geomalgorithms.com/a05-_intersect-1.html
dir = [0; 0; 1];
pz = pt + dir;

l = pz - pt;
l0 = pt;

p0 = P0(1:3);
n = Hn1b2(1:3,3);

% Return results
d = dot(p0 - l0, n)/dot(l, n);
end

== matlab function main/MotionLab Simulator/Simulate Qualisys ==
  data: phi input; pt input; qtm output Bus: ST_QualisysFeedback; l input
function qtm = fcn(phi, pt, l)

data = coder.load('motionlab/calib.mat');
calib = data.calib;

% Get hook position in {n1}
ph = pendel.kinematics(pt, phi, l);

% Transform from {n1} to {g}
Hgq = calib.WORLD_TO_QTM.H;
Hgn = calib.WORLD_TO_EM8000.H;

Hqn = math3d.InvH(Hgq)*Hgn;

Ph = Hqn*[ph; 1];

% Return simulatoin
qtm.d = 60/1000.0;
qtm.x = Ph(1);
qtm.y = Ph(2);
qtm.z = Ph(3);

== matlab function main/WaveSimulator/zyx2xyz1 ==
  data: eta input; eta output
function eta = fcn(eta)

% Convert Angle sequence
eta(4:6) = math3d.zyx2xyz(eta(4:6));

end

== matlab function main/MotionLab Simulator/Feedback Simulator/MruEM8000/MruJacobian ==
  data: eta input; v output; eta_t input
function v = fcn(eta, eta_t)

% Velcoity Jacobian
J = eye(6);
J(4:6,4:6) = math3d.Tphi(eta(4:6), 'xyz');

% Body fixed velocities
v = J\eta_t;

end

== matlab function main/MotionLab Simulator/Feedback Simulator/EM1/Jacobian ==
  data: eta input; v output; eta_t input
function v  = fcn(eta, eta_t)

J = eye(6);

J(4:6,4:6) = math3d.Tphi(eta(4:6), 'xyz');

v = J\eta_t;

== matlab function main/MotionLab Simulator/Feedback Simulator/EM2/Jacobian ==
  data: eta input; v output; eta_t input
function v  = fcn(eta, eta_t)

J = eye(6);

J(4:6,4:6) = math3d.Tphi(eta(4:6), 'xyz');

v = J\eta_t;

== matlab function main/Simulate Measurements ==
  data: x output; mru1 input; comau input; u output; pendulum input; winch input; z output; Kdc output; omega output; zeta output
function [x, u, z, Kdc, omega, zeta] = fcn(mru1, comau, pendulum, winch)

Kdc = winch.Kdc;
omega = winch.omega;
zeta = winch.zeta;

% State vector
eta = [
    mru1.surge
    mru1.sway
    mru1.heave
    mru1.phi
    mru1.theta
    mru1.psi
];

v = [
    mru1.surge_t
    mru1.sway_t
    mru1.heave_t
    mru1.wx
    mru1.wy
    mru1.wz
];

v_t = zeros(6,1);

p = comau.p;
p_t = comau.p_t;
p_tt = comau.p_tt;



phi = pendulum.phi;
phi_t = pendulum.phi_t;
c = pendulum.c;

l = winch.l;
l_t = winch.l_t;

x = [
    eta
    v
    v_t
    p
    p_t
    p_tt
    l
    l_t
    phi
    phi_t
    c
];


% Control input
l_ref = winch.l_ref;

u = [
    l_ref
];

% Measurements
z = observer.h(x);

== matlab function main/EKF ==
  data: Ts input; Q input; R input; u input; x output; z input; Kdc input; omega input; zeta input; x input; P input; P output
function [x, P] = fcn(Ts, Q, R, u, z, Kdc, omega, zeta, x, P)

% Prediction
xPred = observer.f(x, u, Ts, omega, zeta, Kdc);
F = observer.fJacobian(x, u, Ts, omega, zeta, Kdc);
PPred = F*P*F' + Q;

% Measurement update
y = z - observer.h(xPred);

H = observer.hJacobian(xPred);
S = H*PPred*H' + R;

K = PPred*H'*inv(S);


x = xPred + K*y;
I = eye(length(x));
P = (I - K*H)*PPred;


end
